simulink model "Simulation_Robotinos"  (R2017b)
settings: Solver=FixedStepAuto  StartTime=0.0  StopTime=100.0  FixedStep=0.005  RelTol=1e-3
InitFcn:
  | dt=0.005;
libraries: simulink x15
(part 3 of 4)

== matlab function Simulation_Robotinos/Bahnplanung2/Positionen_Robotinos_Filtern ==
  data: UDPDaten input; RobPos output; RobotinoID input; StoerPos output size=[1 15]; altePos input size=[1 15]; altePos1 output size=[1 15]
function [RobPos,StoerPos,altePos1]      = fcn(UDPDaten , RobotinoID, altePos)
StoerPos=zeros([1 15]);
RobPos=zeros([1 3]);
altePos1=zeros([1 15]);
%     case 5
%         RobPos(1:3) = UDPDaten(13:15);
%         StoerPos(1:12)=UDPDaten(1:12);
%Positionmerken
for x=0:4
    temp=abs(UDPDaten((x*3)+1:(x*3)+3));
    test=sum(temp);
    if(test==0)
     altePos1((x*3)+1:(x*3)+3)=altePos((x*3)+1:(x*3)+3);
    else
     altePos1((x*3)+1:(x*3)+3)=UDPDaten((x*3)+1:(x*3)+3);
    end
end

if RobotinoID==5
        RobPos(1:3) = altePos1(13:15);
        StoerPos(1:12)=altePos1(1:12);
    elseif RobotinoID == 4
        RobPos(1:3) = altePos1(10:12);
        StoerPos(1:9)=altePos1(1:9);
        StoerPos(10:12)=altePos1(13:15);
    elseif RobotinoID == 3
        RobPos(1:3) = altePos1(7:9);
        StoerPos(1:6)=altePos1(1:6);
        StoerPos(7:9)=altePos1(10:12);%      StoerPos(7:12)=UDPDaten(10:15);
        StoerPos(10:12)=altePos1(13:15);
    elseif RobotinoID == 2
        RobPos(1:3) = altePos1(4:6);
        StoerPos(1:3)=altePos1(1:3);
        StoerPos(4:9)=altePos1(7:12);%     StoerPos(4:12)=UDPDaten(7:15);
        StoerPos(10:12)=altePos1(13:15);
    elseif RobotinoID == 1
        RobPos(1:3) = altePos1(1:3);
        StoerPos(1:9)=altePos1(4:12);%     StoerPos(1:12)=UDPDaten(4:15);
        StoerPos(10:12)=altePos1(13:15);
        
end

== matlab function Simulation_Robotinos/Bahnplanung2/Status ==
  data: Fehler_IN input; Status_IN input; Status output
function Status       = fcn(Fehler_IN ,Status_IN)
if Fehler_IN > 0 
    Status = Fehler_IN + 4;
else
    Status = Status_IN;
end
end

== matlab function Simulation_Robotinos/Bahnplanung2/Trafo ==
  data: Vektor input; V_RobX output; Winkel input; V_RobY output
function [V_RobX, V_RobY]= fcn(Vektor,Winkel)
V_RobX=(cos(Winkel)*Vektor(1)+sin(Winkel)*Vektor(2));
V_RobY=(cos(Winkel)*Vektor(2)-sin(Winkel)*Vektor(1));

== matlab function Simulation_Robotinos/Bahnplanung2/Vektorberechnung/AusweichVektorBerechnung ==
  data: Zone input; ZielPos input; RobotinoPos input; Ausweichwert input; Vektor_In input; Vektor output
function Vektor  = fcn(Zone,ZielPos,RobotinoPos,Ausweichwert,Vektor_In)
Vektor=zeros([1 2]);
%Ausweichmanöver
Distanz=sqrt((RobotinoPos(1)-ZielPos(1))^2+(RobotinoPos(2)-ZielPos(2))^2);
K=1.4;
AVX=zeros([1 4]);
AVY=zeros([1 4]);
 for x=1:4
 AVX(x)=-K*Ausweichwert(2,x)*cos(Ausweichwert(1,x));
 AVY(x)=-K*Ausweichwert(2,x)*sin(Ausweichwert(1,x));
 end
if (Zone==0) && ((Distanz > 300)&&(RobotinoPos(2)> 500)&&(RobotinoPos(1)> 500))
 VektorX=Vektor_In(1)+sum(AVX);
 VektorY=Vektor_In(2)+sum(AVY);
else
 VektorX=Vektor_In(1);
 VektorY=Vektor_In(2);
end

%Bremsen vor dem Ziel

MaxDis=1000;
if Distanz > MaxDis
Vektor(1) = VektorX;
Vektor(2) = VektorY;
else
Vektor(1) = VektorX*Distanz/MaxDis;
Vektor(2) = VektorY*Distanz/MaxDis;  
end

end

== matlab function Simulation_Robotinos/Bahnplanung2/Vektorberechnung/Ausweichmanoever ==
  data: RobotinoPos input; StoerPos input; Vektor input; Ausweich output
function Ausweich  = fcn(RobotinoPos, StoerPos, Vektor)
Abstand=zeros([2 4]);
Ausweich=zeros([2 4]);%Zeile1 =Richtung(winkel in Rad) Zeile2=Intensität
for i=1:4
    Abstand(1,i)=-RobotinoPos(1)+StoerPos(1+((i-1)*3));
    Abstand(2,i)=-RobotinoPos(2)+StoerPos(2+((i-1)*3));
    Hyp=sqrt(Abstand(1,i)^2+Abstand(2,i)^2);
    if(Hyp==0)
        Hyp=1e-22;
    end
    if Hyp <=1000
        if Abstand(1,i) >= 0
             Ausweich(1,i)=+asin(Abstand(2,i)/Hyp)-pi/2;
        else
            Ausweich(1,i)=-asin(Abstand(2,i)/Hyp)+pi/2;
        end
        HypZiel=sqrt(Vektor(1)^2+Vektor(2)^2);
         if Vektor(1) >= 0
            Fahrwinkel=+asin(Vektor(2)/HypZiel);
        else
            Fahrwinkel=-asin(Vektor(2)/HypZiel)+pi;
        end
        if abs(Fahrwinkel-(Ausweich(1,i)+pi/2))<=pi
            if((Fahrwinkel-(Ausweich(1,i)+pi/2)) <= pi/6) && ((Fahrwinkel-(Ausweich(1,i)+pi/2))  >= -pi/6)
            Ausweich(2,i)=1;
             else
           Ausweich(2,i)=0; 
            end
        else
            if((2*pi)-abs(Fahrwinkel-(Ausweich(1,i)+pi/2)) <= pi/6) 
            Ausweich(2,i)=1;
             else
           Ausweich(2,i)=0; 
            end
        end
%         if (abs(Fahrwinkel)>pi/2) && (RobotinoPos(2)>1600)
%              if abs(Fahrwinkel-(Ausweich(1,i)+pi/2))<=pi
%             if((Fahrwinkel-(Ausweich(1,i)+pi/2)) <= pi/6) && ((Fahrwinkel-(Ausweich(1,i)+pi/2))  >= -pi/6)
%             Ausweich(2,i)=-0.5;
%              else
%            Ausweich(2,i)=0; 
%             end
%         else
%             if((2*pi)-abs(Fahrwinkel-(Ausweich(1,i)+pi/2)) <= pi/6) 
%             Ausweich(2,i)=-0.5;
%              else
%            Ausweich(2,i)=0; 
%             end
%         end
        %end
%         if (Vektor(2)~=0) && (sin(Ausweich(1,i)+pi/2)~=0)
%             Ausweich(2,i)=Vektor(2)/sin(Ausweich(1,i)+pi/2);
%         elseif (Vektor(1)~=0)&&(cos(Ausweich(1,i)+pi/2)~=0)
%              Ausweich(2,i)=Vektor(1)/cos(Ausweich(1,i)+pi/2);
%         else
%              Ausweich(2,i)=0;
%         end
    else
        Ausweich(1,i)=0;
        Ausweich(2,i)=0;
    end
    if StoerPos(2+((i-1)*3))<300
        Ausweich(2,i)=0;
    end
end

== matlab function Simulation_Robotinos/Bahnplanung2/Vektorberechnung/FahrendeRobotinosErkennen ==
  data: Stoerpos input; Robotinofaehrt output; Stoeralt input
function Robotinofaehrt = fcn(Stoerpos,Stoeralt)
Robotinofaehrt=zeros([1 4]);
for x=1:4
    if (abs(Stoeralt(1+(3*(x-1)))-Stoerpos(1+(3*(x-1)))) >= 10) && (abs(Stoeralt(2+(3*(x-1)))-Stoerpos(2+(3*(x-1)))) >= 10)
        Robotinofaehrt(x)=1;
    else
        Robotinofaehrt(x)=0;
    end
end

== matlab function Simulation_Robotinos/Bahnplanung2/Vektorberechnung/IR_Daten_Erfassen ==
  data: RobotinoDaten input; IRWerte output; RobPos input
function IRWerte = fcn(RobotinoDaten,RobPos)
IRWerte=zeros([2 9]);
IRDaten=zeros([1 9]);
IRDaten=RobotinoDaten(6:14);

for x=1:9
    if  (isnan(IRDaten(x))==0) && (IRDaten(x) <= 150)
    IRWerte(1,x)=cos(((x-1)*40*pi/180)+RobPos(3))*(IRDaten(x)+200)+RobPos(1);
    IRWerte(2,x)=sin(((x-1)*40*pi/180)+RobPos(3))*(IRDaten(x)+200)+RobPos(2);
    else
    IRWerte(1,x)=NaN;
    IRWerte(2,x)=NaN;
    end
end

== matlab function Simulation_Robotinos/Bahnplanung2/Vektorberechnung/Vektorberechnung ==
  data: StoerPos input; IRWerte input; RobotinoPos input; RobotinoFaehrt input; ZielPos input; Vektor output; Zone output; AlteZone input
function [Vektor,Zone] = fcn( StoerPos, IRWerte,RobotinoPos,RobotinoFaehrt,ZielPos,AlteZone)
Stationen=[1103,2308,3507,4694,6300,6300;
            2832,2832,2832,2832,2608,3085;];
Vektor=zeros([1 2]);
%Stationen Einflussvektor
K=500;
sigma=187;
SVX=zeros([1 6]);
SVY=zeros([1 6]);
for x=1:4 %%Stationspotentiale
SVX(x)= -K*exp(-((RobotinoPos(1)-Stationen(1,x))^2+(RobotinoPos(2)-Stationen(2,x))^2)/(2*(sigma^2)))*((RobotinoPos(1)-Stationen(1,x))/(sigma^2));
SVY(x)= -K*exp(-((RobotinoPos(1)-Stationen(1,x))^2+(RobotinoPos(2)-Stationen(2,x))^2)/(2*(sigma^2)))*((RobotinoPos(2)-Stationen(2,x))/(sigma^2));
end
K=300;
sigma=100; %% mal schauen ob so gut
for x=5:6 %% Ladestation
SVX(x)= -K*exp(-((RobotinoPos(1)-Stationen(1,x))^2+(RobotinoPos(2)-Stationen(2,x))^2)/(2*(sigma^2)))*((RobotinoPos(1)-Stationen(1,x))/(sigma^2));
SVY(x)= -K*exp(-((RobotinoPos(1)-Stationen(1,x))^2+(RobotinoPos(2)-Stationen(2,x))^2)/(2*(sigma^2)))*((RobotinoPos(2)-Stationen(2,x))/(sigma^2));
end
%Zielvektor
K=0.7;%=0.5;
if (RobotinoPos(1)~=ZielPos(1)) && (RobotinoPos(2)~=ZielPos(2))  %%Ziel
    ZVX = K*(RobotinoPos(1)-ZielPos(1))/sqrt((RobotinoPos(1)-ZielPos(1))^2 +(RobotinoPos(2)-ZielPos(2))^2);
    ZVY = K*(RobotinoPos(2)-ZielPos(2))/sqrt((RobotinoPos(1)-ZielPos(1))^2 +(RobotinoPos(2)-ZielPos(2))^2);
else
    ZVX=0;
    ZVY=0;
end

%Robtino Stoervektoren
%K=25 im Fifo

RVX=zeros([1 4]);
RVY=zeros([1 4]);
for x=1:4
if (RobotinoFaehrt(x) == 1) && (RobotinoPos(2)> 500)
K=1300;%K=1000;
sigma=240;
elseif (RobotinoPos(2)> 2500)
K=700;%500
sigma=200;
elseif (RobotinoPos(2)< 2500)
K=1000;%700
sigma=200;
end
RVX(x)=-K*exp(-((RobotinoPos(1)-StoerPos((x*3)-2))^2+(RobotinoPos(2)-StoerPos((x*3)-1))^2)/(2*(sigma^2)))*((RobotinoPos(1)-StoerPos((x*3)-2))/(sigma^2));
RVY(x)=-K*exp(-((RobotinoPos(1)-StoerPos((x*3)-2))^2+(RobotinoPos(2)-StoerPos((x*3)-1))^2)/(2*(sigma^2)))*((RobotinoPos(2)-StoerPos((x*3)-1))/(sigma^2));
end

%Infrarot Einflussvektor
K=600;%500;
sigma=250;
IRVX=zeros([1 9]);
IRVY=zeros([1 9]);
for x=1:9
    if(isnan(IRWerte(1,x))==0)||(isnan(IRWerte(2,x))==0)
       if (RobotinoPos(2)> 500)
    IRVX(x)=-K*exp(-((RobotinoPos(1)-IRWerte(1,x))^2+(RobotinoPos(2)-IRWerte(2,x))^2)/(2*(sigma^2)))*((RobotinoPos(1)-IRWerte(1,x))/(sigma^2));
    IRVY(x)=-K*exp(-((RobotinoPos(1)-IRWerte(1,x))^2+(RobotinoPos(2)-IRWerte(2,x))^2)/(2*(sigma^2)))*((RobotinoPos(2)-IRWerte(2,x))/(sigma^2));
       else
    IRVX=0;
    IRVY=0;
       end
    else
    IRVX(x)=0;
    IRVY(x)=0;
    end
end


 
K=0.4; %Steigung der schrägen
x=RobotinoPos(1);
y=RobotinoPos(2);
x_test=0;
y_test=0;
VektorX=0;
VektorY=0;
%% Einteilung des Vektorbereichs in verschidene Zonen
%%Einbahnstraßen hinter und neben den Stationen
 if (x >601) && (x<=5301) && (y>2501) && (y<=3201)
    Zone=4;
elseif (x >2751) && (x<=5501) && (y>3201)
    Zone=1;
elseif (x > 601) && (x<=2751) && (y>3201)
    Zone=2;
 elseif (x<=601) && (y>2001)%% y auf 2001 von 2501
     Zone=3;  
 elseif (x >5001) && (y>2501) && (AlteZone==1 || AlteZone==5)
     Zone=5;
 else
     Zone=0;
 end

KE=1000;
sigma=50;
Parabel=1000;
 if Zone == 0 % Fahrbereich
     if (x <= 5500) && (y <= 2500)
         x_test=(1/sigma)*KE*exp(-x/sigma);
         y_test=(-1/sigma)*KE*exp((y-2500)/sigma);
     elseif (x > 5500) && (y <= 2500)
         x_test=(1/sigma)*KE*exp((-(x-5500)+(y-2500))/sigma);
         y_test=(-1/sigma)*KE*exp((-(x-5500)+(y-2500))/sigma);
     elseif (x > 5500) && (y > 2500)
         x_test=(1/sigma)*KE*exp(-(x-5500)/sigma);
         y_test=(-1/sigma)*KE*exp((y-3600)/sigma);
     end
 MVX=x_test+(-1/sigma)*KE*exp((x-7400)/sigma);
 MVY=y_test+(1/sigma)*KE*exp(-y/sigma);
 
 VektorX=sum(SVX(5:6))+sum(RVX)+ZVX+sum(IRVX)-MVX;
 VektorY=sum(SVY(5:6))+sum(RVY)+ZVY+sum(IRVY)-MVY;
 elseif Zone == 1 %Rinne nach rechts weg
     MVX=K; %Konstante Steigung
     MVY=-2*(y-3500)/Parabel; % Parabel abgeleitet
 VektorX=sum(RVX)-MVX;
 VektorY=sum(RVY)-MVY;
 elseif Zone == 2 %Rinne nach links weg
     MVX=-K; %Konstante Steigung
     MVY=-2*(y-3500)/Parabel; % Parabel abgeleitet
      VektorX=sum(RVX)-MVX;
      VektorY=sum(RVY)-MVY;
 elseif Zone == 3 %Rinne nach unten weg
     MVX=-2*(x-300)/Parabel; %Konstante Steigung
     MVY=-K; % Parabel abgeleitet
     VektorX=sum(RVX)+sum(IRVX)-MVX;
     VektorY=sum(RVY)+sum(IRVY)-MVY;
 elseif Zone == 5 %Rinne vorne weg
     MVX=-2*(x-5500)/Parabel; %Konstante Steigung
     MVY=-K; % Parabel abgeleitet
     VektorX=sum(RVX)+sum(IRVX)-MVX;
     VektorY=sum(RVY)+sum(IRVY)-MVY;
 else 
     MVX=0;
     MVY=K;
      VektorX=sum(RVX)+sum(SVX(1:4))-MVX;
      VektorY=sum(RVY)+sum(SVY(1:4))-MVY;
 end  
      Vektor(1)=VektorX;
      Vektor(2)=VektorY;
 end

== matlab function Simulation_Robotinos/Bahnplanung2/Vektorbrbegrenzungberchnen1 ==
  data: Vektor_In input; IRDaten input; Vektor output; Transportbereich_aktiv input; RobPos input; FilterIN input; Filter output
function [Vektor,Filter] = fcn(Vektor_In,IRDaten,Transportbereich_aktiv,RobPos,FilterIN)
Vektor=zeros([1 2]);
Filter=zeros([10 2]);
if (Transportbereich_aktiv==1) && (RobPos(1)>=0) && (RobPos(2)>=0)
    

 Filter(1,1)=Vektor_In(1);
 Filter(1,2)=Vektor_In(2);
 for x=1:9
     Filter(x+1,1)=FilterIN(x,1);
     Filter(x+1,2)=FilterIN(x,2);     
 end
 Vektor(1) =sum(Filter(:,1))/10;
 Vektor(2) =sum(Filter(:,2))/10;
 
 %Vektor(1) = Vektor_In(1);
 %Vektor(2) = Vektor_In(2);
 for x=1:9
if  (isnan(IRDaten(1,x))==0) && (IRDaten(1,x) <= 150)
    for x=1:2
    K=0.1; %Begrenzung langsame Zone
        if  Vektor(x)> K
            Vektor(x) = K;
        elseif Vektor(x) <-K
            Vektor(x)=-K;
        end
    end
end
 end
if (RobPos(2)<500)||(RobPos(2)>2300)
    for x=1:2
    K=0.3; %Begrenzung langsame Zone
        if  Vektor(x)> K
            Vektor(x) = K;
        elseif Vektor(x) <-K
            Vektor(x)=-K;
        end
    end
else
    for x=1:2
    K=0.7; %Begrenzung schnelle Zone
        if  Vektor(x)> K
            Vektor(x) = K;
        elseif Vektor(x) <-K
            Vektor(x)=-K;
        end
    end
end
end

== stateflow chart Simulation_Robotinos/Bahnplanung3/Auftrags_Koordination ==
  settings: updateMethod=DISCRETE  sampleTime=dt
  state Auftragskoordination
    state WerkstueckAufgenommen
      entry:Werkstueck=1,
      AktuellesZiel=ZielPos,
      Bearbeitet=1;
    state WerkstueckAbgelegt
      entry:Werkstueck=0,
      AktuellesZiel=ZielPos,
      Bearbeitet=1;
    state KeinWerkstueckAufgenommen
      entry:Werkstueck=0,
      AktuellesZiel=WerkstueckPos,
      Bearbeitet=1;
    state AufAuftragWarten
      entry:Werkstueck=0,
      AktuellesZiel=100
      Bearbeitet=0;
    state Laden
      entry:Werkstueck=0,
      AktuellesZiel=90,
      Bearbeitet=1;
    state Ladenabgeschlossen
      entry:Werkstueck=0,
      AktuellesZiel=90,
      Bearbeitet=1;
    WerkstueckAufgenommen -> WerkstueckAufgenommen [order 1] : [Fehler==3]
    WerkstueckAufgenommen -> WerkstueckAbgelegt [order 3] : [Werkstueckerkannt==0 && Transportbereich==0]
    KeinWerkstueckAufgenommen -> WerkstueckAufgenommen [order 1] : [Werkstueckerkannt==1 && Transportbereich==1]
    WerkstueckAufgenommen -> AufAuftragWarten [order 2] : [Fehler==2  && Transportbereich==1]
    (default) -> AufAuftragWarten
    WerkstueckAbgelegt -> AufAuftragWarten : [Werkstueckerkannt==0 && Transportbereich==1]
    KeinWerkstueckAufgenommen -> AufAuftragWarten [order 2] : [Fehler==1&& Transportbereich==1]
    AufAuftragWarten -> KeinWerkstueckAufgenommen [order 1] : [NeuerAuftrag ==1 && WerkstueckPos< 80 && Fehler==0]
    AufAuftragWarten -> Laden [order 2] : [NeuerAuftrag ==1 && WerkstueckPos>= 80]
    Ladenabgeschlossen -> AufAuftragWarten : [Transportbereich==1]
    Laden -> Ladenabgeschlossen : [Status==4]
  data: NeuerAuftrag input; WerkstueckPos input; ZielPos input; AktuellesZiel output; Werkstueck output; Werkstueckerkannt input; Transportbereich input; Bearbeitet output; Status input; Fehler input

== matlab function Simulation_Robotinos/Bahnplanung3/Fehler_Merker ==
  data: Fehler_IN input; Reset input; Transportbereich input; Werkstueckerkannt input; Werkstueck input; Fehler_OUT output; Fehler_alt input
function Fehler_OUT       = fcn(Fehler_IN ,Reset, Transportbereich, Werkstueckerkannt,Werkstueck, Fehler_alt)
if Reset == 1 || Fehler_IN ~= 0
    Fehler_OUT=Fehler_IN;
else
    if Transportbereich == 1 && Werkstueckerkannt~=1 && Werkstueck == 1
        Fehler_OUT = 2;
    else
       Fehler_OUT=Fehler_alt; 
    end 
end
end

== stateflow chart Simulation_Robotinos/Bahnplanung3/Fifo Steuerung/Fifo ==
  settings: updateMethod=DISCRETE  sampleTime=dt
  state FIFOStationen
    state Auftrag_Roboter_1
    state Zielbereich_untersuchen
      entry:
      ersterFifo=floor(Zielstation/2)*3+2*mod(Zielstation,2)+1;
    state Fifo_doppelt_besetzt
      entry:
      dritterFifo=floor(Zielstation/2)*3+2-2*mod(Zielstation,2)+1,
      Fifo=3;
    state Fifo_einfachbesetzt1
      entry:
      zweiterFifo=floor(Zielstation/2)*3+1+1,
      Fifo=2;
    state Fifo_voll
      entry:
      Fifo=4;
    state Fifo_frei
      entry:
      Fifo=1;
    state Uebergabepunkt_gleich_Zielpunkt
      entry:
      Fifo=0;
    (default) -> Auftrag_Roboter_1
    Auftrag_Roboter_1 -> Zielbereich_untersuchen : [Zielposition>-1]
    Zielbereich_untersuchen -> Fifo_einfachbesetzt1 [order 1] : [(FifoArray(ersterFifo)~=0)| (FifoArray(ersterFifo)==0 & StationArray(Zielstation+1)~=0) ]
    Uebergabepunkt_gleich_Zielpunkt -> Zielbereich_untersuchen
    Zielbereich_untersuchen -> Uebergabepunkt_gleich_Zielpunkt [order 2]
    Fifo_einfachbesetzt1 -> Fifo_doppelt_besetzt [order 1] : [(FifoArray(zweiterFifo)~=0)]
    Fifo_doppelt_besetzt -> Fifo_voll [order 2] : [(FifoArray(dritterFifo)~=0)]
    Fifo_einfachbesetzt1 -> Fifo_frei [order 2] : [FifoArray(ersterFifo)==0]
    Fifo_frei -> Uebergabepunkt_gleich_Zielpunkt : [ StationArray(Zielstation+1)==0]
    Fifo_doppelt_besetzt -> Fifo_einfachbesetzt1 [order 1] : [FifoArray(zweiterFifo)==0]
    Fifo_voll -> Fifo_doppelt_besetzt : [FifoArray(dritterFifo)==0]
  state Wartebereich
    entry: Fifo=4;
  state Ladestation
    entry: Fifo=0;
  state Ladestation1
    entry: Fifo=4;
  FIFOStationen -> FIFOStationen [order 1] : [after(10000, tick)]
  (default) -> Wartebereich
  Wartebereich -> FIFOStationen [order 1] : [Zielstation<8]
  FIFOStationen -> Wartebereich [order 2] : [Zielstation==10]
  Ladestation -> Wartebereich [order 1] : [Zielstation==10]
  Wartebereich -> Ladestation [order 2] : [Zielstation>=8 & Zielstation<10]
  Ladestation -> FIFOStationen [order 2] : [Zielstation<8]
  FIFOStationen -> Ladestation [order 3] : [Zielstation>=8 & Zielstation<10]
  Ladestation -> Ladestation1 [order 3] : [Ladenarray(1)~=0]
  Ladestation1 -> Ladestation : [Ladenarray(1)==0]
  data: FifoArray input; Zielposition input; Zielstation input; Fifo output; StationArray input; dritterFifo local; zweiterFifo local; ersterFifo local; Ladenarray input

== matlab function Simulation_Robotinos/Bahnplanung3/Fifo Steuerung/Globale Markierung1 ==
  data: StationArray1 output; Robbi input; FifoArray input; FifoArray1 output; LadeArray1 output; LadeArray input
function [StationArray1,FifoArray1,LadeArray1]= fcn(Robbi,FifoArray,LadeArray)
X=zeros([1 4]);
Y=zeros([1 4]);
X=[Robbi(1) Robbi(4) Robbi(7) Robbi(10)];
Y=[Robbi(2) Robbi(5) Robbi(8) Robbi(11)];
FifoArray1=zeros([1 12]);
FifoArray1=FifoArray(1:12);
StationArray1=zeros([1 8]);
LadeArray1=zeros([1 2]);
LadeArray1=LadeArray(1:2);
N=zeros([1 4]);
S=zeros([1 4]);
L=zeros([1 4]);
  for n= 1 : 1 : 4
    L(n)=round((Y(n)-2592)/500)+1;
    N(n)=round((X(n)-703)/425)+1;   % Berechnung in welchem Fifo der Roboter sich befindet
    S(n)=round((X(n)-900)/560)+1;   %Berechnung in welcher Station der Roboter sich befindet
     if (X(n)<=6000 || X(n)>6500)
        for i=1:2
            if LadeArray1(i)==n
                LadeArray1(i)=0;
            end
        end
     end
    if (X(n)>6000 && X(n)<=6500 && Y(n)>2300 && Y(n)<=3300 && L(n)<=2 && L(n)>0)
        LadeArray1(1)=n;
        LadeArray1(2)=n;
    end  
   
    for i=1:8
          if StationArray1(i)==n
                StationArray1(i)=0;
          end
    end
    if (Y(n)>2000 && Y(n)<3300 && X(n)<5100 && S(n)<=8 && S(n)>0) %% Setzen der Stationspos.
         for i=1:12
            if FifoArray1(i)==n
                FifoArray1(i)=0;
            end
         end
       
        StationArray1(S(n))=n;
    end
    if (Y(n)<450 && X(n)>100 && X(n)<6000 && N(n)<=12 && N(n)>0) %% Setzten der aktuellen Fifo Pos
        for i=1:12
            if FifoArray1(i)==n
                FifoArray1(i)=0;
            end
        end
            FifoArray1(N(n))=n;
    end  
    if (X(n)>6000 && Y(n)<2000)%%Rücksetzen de4r FIFOs auf Warteposition
        for i=1:12
            if FifoArray1(i)==n
                FifoArray1(i)=0;
            end
        end
    end
  end
end

== matlab function Simulation_Robotinos/Bahnplanung3/Fifo Steuerung/Positionszuweisung ==
  data: Fifo input; Zielstation input; Endposition output; RoboterID input
function Endposition = fcn(Fifo,Zielstation,RoboterID)
Endposition=zeros([1 2]);

WartepositionX= [6200 6800 7200 7200 7200]; %[7200 6800 7200 6200 7200];
WartepositionY= [250 250 550 1150 1750];    %[550 250 1150 250 1750];

StationvorneX=[853 1361 2058 2559 3256 3762 4448 4953 5965 5965];
StationvorneY=[2300 2300 2300 2300 2300 2300 2300 2300 3080 2593];
%Stationhinten=[856 1364 2059 2560 3259 3763 4451 4958];

ersterFifo=floor(Zielstation/2)*3+2*mod(Zielstation,2);
zweiterFifo=floor(Zielstation/2)*3+1;
dritterFifo=floor(Zielstation/2)*3+2-2*mod(Zielstation,2);

if Fifo==0
    Endposition(1)=StationvorneX(Zielstation+1);
    Endposition(2)=StationvorneY(Zielstation+1);
    else if Fifo==1
        Endposition(1)= ersterFifo*425+703;
        Endposition(2)= 250;
       
    else if Fifo==2
            Endposition(1)= zweiterFifo*425+703;
            Endposition(2)= 250;
        
    else if Fifo==3
            Endposition(1)= dritterFifo*425+703;
            Endposition(2)= 250;
            else
            Endposition(2)= WartepositionY(RoboterID);
            Endposition(1)= WartepositionX(RoboterID);
        end
        end
        end
end
end

== matlab function Simulation_Robotinos/Bahnplanung3/Fifo Steuerung/ZielPosSplitten ==
  data: AktuellesZiel input; ZielPos output; Zielstation output
function [ZielPos,Zielstation]= fcn(AktuellesZiel)
ZielPos=mod(AktuellesZiel,10);
Zielstation=round(AktuellesZiel/10);

== matlab function Simulation_Robotinos/Bahnplanung3/Fifo Steuerung/ZielStation_Erreicht ==
  data: Erreicht output; AktuellePos input; Zielpos input
function Erreicht = fcn(AktuellePos,Zielpos)
Abstand=sqrt((AktuellePos(1)-Zielpos(1))^2+(AktuellePos(2)-Zielpos(2))^2);
%S=round((X-900)/560);
if AktuellePos(2) >2000 && Abstand < 150
    Erreicht=1;
else
    Erreicht=0;
end
end

== stateflow chart Simulation_Robotinos/Bahnplanung3/Kommunikation_mit_GW1_3 ==
  settings: updateMethod=DISCRETE  sampleTime=dt
  state KommunikationGW3
    state Fertigungsbereich
      entry:Transportbereich=0,
      Fertigungsbereich=1;
      state RFID_einchecken
        entry:Zielposition=Ziel-mod(Ziel,10)+3,
        Aktion_an_Position=Aktion_Warten,
        Status=2;
      state Startpunkt
        entry: Zielposition=Ziel-mod(Ziel,10);
        Aktion_an_Position=Aktion_Warten,
        Status=1;
      state Warten
        during: Bereich_Verlassen=1,
      state Bereich_verlassen_hinten
        entry:Zielposition=Ziel-mod(Ziel,10)+4,
        Aktion_an_Position=Aktion_Warten,
        Status=1;
      state Bereich_verlassen_vorne1
        entry:Zielposition=Ziel-mod(Ziel,10),
        Aktion_an_Position=Aktion_Warten,
        Status=1;
      state Warten1
      state Bereich_verlassen
        entry:
        ersterFifo=floor(floor(Ziel/10)/2)*3+2*mod(floor(Ziel/10),2)+1;
        Aktion_an_Position=Aktion_Warten,
      state Position_anfahren
        entry:Zielposition=Ziel,
        Status=1,
        if Werkstueck==0
        Aktion_an_Position=Aktion_Aufnehmen;
        else
        Aktion_an_Position=Aktion_Ablegen;
        end
      state RFID_auschecken
        entry:Zielposition=Ziel-mod(Ziel,10)+3,
        Aktion_an_Position=Aktion_Warten,
        Status=3;
      state Warten2
      Startpunkt -> Startpunkt [order 1] : [Fehler==3]
      (default) -> Startpunkt
      Startpunkt -> RFID_einchecken [order 2] : [Ziel_anfordern==1 & Werkstueck==1]
      Position_anfahren -> Startpunkt [order 3] : [Fehler==3 & Ziel_anfordern==1]
      Startpunkt -> Position_anfahren [order 3] : [Ziel_anfordern==1 & Werkstueck==0]
      RFID_einchecken -> Warten1 : [Ziel_anfordern==1 ]
      Bereich_verlassen_hinten -> Warten : [Ziel_anfordern==1]
      Bereich_verlassen_vorne1 -> Warten : [Ziel_anfordern==1]
      Warten1 -> Position_anfahren : [RFID_Anmeldung==1]
      Bereich_verlassen -> Bereich_verlassen_hinten [order 2]
      Bereich_verlassen -> Bereich_verlassen_vorne1 [order 1] : [FifoArray(ersterFifo)==0]
      Position_anfahren -> Bereich_verlassen [order 2] : [Fehler==1 & Ziel_anfordern==1]
      Position_anfahren -> Bereich_verlassen [order 1] : [Ziel_anfordern==1 & (Aktion_an_Position==Aktion_Ablegen)]
      Warten2 -> Bereich_verlassen : [RFID_Abmeldung==1]
      Position_anfahren -> RFID_auschecken [order 4] : [Ziel_anfordern==1 & (Aktion_an_Position==Aktion_Aufnehmen) & Fehler==0]
      RFID_auschecken -> Warten2 : [Ziel_anfordern==1]
    state Ladestationanfahren2
      entry: Zielposition=100,
      Transportbereich=0,
      Fertigungsbereich=1,
      Status=1;
    state Transportbereich
      entry:Transportbereich=1,
      Zielposition=999,
      Fertigungsbereich=0,
      Bereich_Verlassen=0,
      Geladen=0,
      Status=1;
    state Warten3
    state Ladestationanfahren1
      entry: Zielposition=80,
      Transportbereich=0,
      Fertigungsbereich=1,
      Status=1;
    state Laden4
      entry: Zielposition=110,
      Transportbereich=0,
      Fertigungsbereich=1,
      Geladen=1,
      Status=4;
    state Laden2
      entry: Zielposition=110,
      Transportbereich=0,
      Fertigungsbereich=1,
      Status=1;
    state Laden1
      entry: Zielposition=90,
      Transportbereich=0,
      Fertigungsbereich=1,
      Status=1;
    state Laden3
      entry: Zielposition=90,
      Transportbereich=0,
      Fertigungsbereich=1,
      Geladen =1,
      Status=4;
    (default) -> Transportbereich
    Ladestationanfahren2 -> Transportbereich [order 2] : [ Geladen==1 & Ziel_anfordern==1 ]
    Transportbereich -> Fertigungsbereich [order 1] : [(ZielStation_Erreicht==1) & (floor(Ziel/10)<=7)]
    Transportbereich -> Ladestationanfahren2 [order 2] : [(ZielStation_Erreicht==1) & (floor(Ziel/10)==9)]
    Warten3 -> Transportbereich
    Fertigungsbereich -> Warten3 : [Bereich_Verlassen==1]
    Ladestationanfahren2 -> Laden2 [order 1] : [ Geladen==0 & Ziel_anfordern==1 ]
    Laden4 -> Ladestationanfahren2 : [Ladenabgeschlossen==1 ]
    Transportbereich -> Ladestationanfahren1 [order 3] : [(ZielStation_Erreicht==1) & (floor(Ziel/10)==8)]
    Ladestationanfahren1 -> Transportbereich [order 2] : [ Geladen==1 & Ziel_anfordern==1 ]
    Ladestationanfahren1 -> Laden1 [order 1] : [ Geladen==0 & Ziel_anfordern==1 ]
    Laden3 -> Ladestationanfahren1 : [Ladenabgeschlossen==1 ]
    Laden2 -> Laden4 : [Ziel_anfordern==1 ]
    Laden1 -> Laden3 : [Ziel_anfordern==1 ]
  data: Transportbereich output; Fertigungsbereich output; Ziel input; Zielposition output; Aktion_an_Position output double; Aktion_Warten local double =0; Aktion_Aufnehmen local double =1; Aktion_Ablegen local double =2; Werkstueck input double; Bereich_Verlassen local; Status output; FifoArray input; ersterFifo local double; Ziel_anfordern input; ZielStation_Erreicht input double; RFID_Anmeldung input; RFID_Abmeldung input; Ladenabgeschlossen input; Geladen local; Fehler input

== matlab function Simulation_Robotinos/Bahnplanung3/Positionen_Robotinos_Filtern ==
  data: UDPDaten input; RobPos output; RobotinoID input; StoerPos output size=[1 15]; altePos input size=[1 15]; altePos1 output size=[1 15]
function [RobPos,StoerPos,altePos1]      = fcn(UDPDaten , RobotinoID, altePos)
StoerPos=zeros([1 15]);
RobPos=zeros([1 3]);
altePos1=zeros([1 15]);
%     case 5
%         RobPos(1:3) = UDPDaten(13:15);
%         StoerPos(1:12)=UDPDaten(1:12);
%Positionmerken
for x=0:4
    temp=abs(UDPDaten((x*3)+1:(x*3)+3));
    test=sum(temp);
    if(test==0)
     altePos1((x*3)+1:(x*3)+3)=altePos((x*3)+1:(x*3)+3);
    else
     altePos1((x*3)+1:(x*3)+3)=UDPDaten((x*3)+1:(x*3)+3);
    end
end

if RobotinoID==5
        RobPos(1:3) = altePos1(13:15);
        StoerPos(1:12)=altePos1(1:12);
    elseif RobotinoID == 4
        RobPos(1:3) = altePos1(10:12);
        StoerPos(1:9)=altePos1(1:9);
        StoerPos(10:12)=altePos1(13:15);
    elseif RobotinoID == 3
        RobPos(1:3) = altePos1(7:9);
        StoerPos(1:6)=altePos1(1:6);
        StoerPos(7:9)=altePos1(10:12);%      StoerPos(7:12)=UDPDaten(10:15);
        StoerPos(10:12)=altePos1(13:15);
    elseif RobotinoID == 2
        RobPos(1:3) = altePos1(4:6);
        StoerPos(1:3)=altePos1(1:3);
        StoerPos(4:9)=altePos1(7:12);%     StoerPos(4:12)=UDPDaten(7:15);
        StoerPos(10:12)=altePos1(13:15);
    elseif RobotinoID == 1
        RobPos(1:3) = altePos1(1:3);
        StoerPos(1:9)=altePos1(4:12);%     StoerPos(1:12)=UDPDaten(4:15);
        StoerPos(10:12)=altePos1(13:15);
        
end

== matlab function Simulation_Robotinos/Bahnplanung3/Status ==
  data: Fehler_IN input; Status_IN input; Status output
function Status       = fcn(Fehler_IN ,Status_IN)
if Fehler_IN > 0 
    Status = Fehler_IN + 4;
else
    Status = Status_IN;
end
end

== matlab function Simulation_Robotinos/Bahnplanung3/Trafo ==
  data: Vektor input; V_RobX output; Winkel input; V_RobY output
function [V_RobX, V_RobY]= fcn(Vektor,Winkel)
V_RobX=(cos(Winkel)*Vektor(1)+sin(Winkel)*Vektor(2));
V_RobY=(cos(Winkel)*Vektor(2)-sin(Winkel)*Vektor(1));

== matlab function Simulation_Robotinos/Bahnplanung3/Vektorberechnung/AusweichVektorBerechnung ==
  data: Zone input; ZielPos input; RobotinoPos input; Ausweichwert input; Vektor_In input; Vektor output
function Vektor  = fcn(Zone,ZielPos,RobotinoPos,Ausweichwert,Vektor_In)
Vektor=zeros([1 2]);
%Ausweichmanöver
Distanz=sqrt((RobotinoPos(1)-ZielPos(1))^2+(RobotinoPos(2)-ZielPos(2))^2);
K=1.4;
AVX=zeros([1 4]);
AVY=zeros([1 4]);
 for x=1:4
 AVX(x)=-K*Ausweichwert(2,x)*cos(Ausweichwert(1,x));
 AVY(x)=-K*Ausweichwert(2,x)*sin(Ausweichwert(1,x));
 end
if (Zone==0) && ((Distanz > 300)&&(RobotinoPos(2)> 500)&&(RobotinoPos(1)> 500))
 VektorX=Vektor_In(1)+sum(AVX);
 VektorY=Vektor_In(2)+sum(AVY);
else
 VektorX=Vektor_In(1);
 VektorY=Vektor_In(2);
end

%Bremsen vor dem Ziel

MaxDis=1000;
if Distanz > MaxDis
Vektor(1) = VektorX;
Vektor(2) = VektorY;
else
Vektor(1) = VektorX*Distanz/MaxDis;
Vektor(2) = VektorY*Distanz/MaxDis;  
end

end

== matlab function Simulation_Robotinos/Bahnplanung3/Vektorberechnung/Ausweichmanoever ==
  data: RobotinoPos input; StoerPos input; Vektor input; Ausweich output
function Ausweich  = fcn(RobotinoPos, StoerPos, Vektor)
Abstand=zeros([2 4]);
Ausweich=zeros([2 4]);%Zeile1 =Richtung(winkel in Rad) Zeile2=Intensität
for i=1:4
    Abstand(1,i)=-RobotinoPos(1)+StoerPos(1+((i-1)*3));
    Abstand(2,i)=-RobotinoPos(2)+StoerPos(2+((i-1)*3));
    Hyp=sqrt(Abstand(1,i)^2+Abstand(2,i)^2);
    if(Hyp==0)
        Hyp=1e-22;
    end
    if Hyp <=1000
        if Abstand(1,i) >= 0
             Ausweich(1,i)=+asin(Abstand(2,i)/Hyp)-pi/2;
        else
            Ausweich(1,i)=-asin(Abstand(2,i)/Hyp)+pi/2;
        end
        HypZiel=sqrt(Vektor(1)^2+Vektor(2)^2);
         if Vektor(1) >= 0
            Fahrwinkel=+asin(Vektor(2)/HypZiel);
        else
            Fahrwinkel=-asin(Vektor(2)/HypZiel)+pi;
        end
        if abs(Fahrwinkel-(Ausweich(1,i)+pi/2))<=pi
            if((Fahrwinkel-(Ausweich(1,i)+pi/2)) <= pi/6) && ((Fahrwinkel-(Ausweich(1,i)+pi/2))  >= -pi/6)
            Ausweich(2,i)=1;
             else
           Ausweich(2,i)=0; 
            end
        else
            if((2*pi)-abs(Fahrwinkel-(Ausweich(1,i)+pi/2)) <= pi/6) 
            Ausweich(2,i)=1;
             else
           Ausweich(2,i)=0; 
            end
        end
%         if (abs(Fahrwinkel)>pi/2) && (RobotinoPos(2)>1600)
%              if abs(Fahrwinkel-(Ausweich(1,i)+pi/2))<=pi
%             if((Fahrwinkel-(Ausweich(1,i)+pi/2)) <= pi/6) && ((Fahrwinkel-(Ausweich(1,i)+pi/2))  >= -pi/6)
%             Ausweich(2,i)=-0.5;
%              else
%            Ausweich(2,i)=0; 
%             end
%         else
%             if((2*pi)-abs(Fahrwinkel-(Ausweich(1,i)+pi/2)) <= pi/6) 
%             Ausweich(2,i)=-0.5;
%              else
%            Ausweich(2,i)=0; 
%             end
%         end
        %end
%         if (Vektor(2)~=0) && (sin(Ausweich(1,i)+pi/2)~=0)
%             Ausweich(2,i)=Vektor(2)/sin(Ausweich(1,i)+pi/2);
%         elseif (Vektor(1)~=0)&&(cos(Ausweich(1,i)+pi/2)~=0)
%              Ausweich(2,i)=Vektor(1)/cos(Ausweich(1,i)+pi/2);
%         else
%              Ausweich(2,i)=0;
%         end
    else
        Ausweich(1,i)=0;
        Ausweich(2,i)=0;
    end
    if StoerPos(2+((i-1)*3))<300
        Ausweich(2,i)=0;
    end
end

== matlab function Simulation_Robotinos/Bahnplanung3/Vektorberechnung/FahrendeRobotinosErkennen ==
  data: Stoerpos input; Robotinofaehrt output; Stoeralt input
function Robotinofaehrt = fcn(Stoerpos,Stoeralt)
Robotinofaehrt=zeros([1 4]);
for x=1:4
    if (abs(Stoeralt(1+(3*(x-1)))-Stoerpos(1+(3*(x-1)))) >= 10) && (abs(Stoeralt(2+(3*(x-1)))-Stoerpos(2+(3*(x-1)))) >= 10)
        Robotinofaehrt(x)=1;
    else
        Robotinofaehrt(x)=0;
    end
end

== matlab function Simulation_Robotinos/Bahnplanung3/Vektorberechnung/IR_Daten_Erfassen ==
  data: RobotinoDaten input; IRWerte output; RobPos input
function IRWerte = fcn(RobotinoDaten,RobPos)
IRWerte=zeros([2 9]);
IRDaten=zeros([1 9]);
IRDaten=RobotinoDaten(6:14);

for x=1:9
    if  (isnan(IRDaten(x))==0) && (IRDaten(x) <= 150)
    IRWerte(1,x)=cos(((x-1)*40*pi/180)+RobPos(3))*(IRDaten(x)+200)+RobPos(1);
    IRWerte(2,x)=sin(((x-1)*40*pi/180)+RobPos(3))*(IRDaten(x)+200)+RobPos(2);
    else
    IRWerte(1,x)=NaN;
    IRWerte(2,x)=NaN;
    end
end

== matlab function Simulation_Robotinos/Bahnplanung3/Vektorberechnung/Vektorberechnung ==
  data: StoerPos input; IRWerte input; RobotinoPos input; RobotinoFaehrt input; ZielPos input; Vektor output; Zone output; AlteZone input
function [Vektor,Zone] = fcn( StoerPos, IRWerte,RobotinoPos,RobotinoFaehrt,ZielPos,AlteZone)
Stationen=[1103,2308,3507,4694,6300,6300;
            2832,2832,2832,2832,2608,3085;];
Vektor=zeros([1 2]);
%Stationen Einflussvektor
K=500;
sigma=187;
SVX=zeros([1 6]);
SVY=zeros([1 6]);
for x=1:4 %%Stationspotentiale
SVX(x)= -K*exp(-((RobotinoPos(1)-Stationen(1,x))^2+(RobotinoPos(2)-Stationen(2,x))^2)/(2*(sigma^2)))*((RobotinoPos(1)-Stationen(1,x))/(sigma^2));
SVY(x)= -K*exp(-((RobotinoPos(1)-Stationen(1,x))^2+(RobotinoPos(2)-Stationen(2,x))^2)/(2*(sigma^2)))*((RobotinoPos(2)-Stationen(2,x))/(sigma^2));
end
K=300;
sigma=100; %% mal schauen ob so gut
for x=5:6 %% Ladestation
SVX(x)= -K*exp(-((RobotinoPos(1)-Stationen(1,x))^2+(RobotinoPos(2)-Stationen(2,x))^2)/(2*(sigma^2)))*((RobotinoPos(1)-Stationen(1,x))/(sigma^2));
SVY(x)= -K*exp(-((RobotinoPos(1)-Stationen(1,x))^2+(RobotinoPos(2)-Stationen(2,x))^2)/(2*(sigma^2)))*((RobotinoPos(2)-Stationen(2,x))/(sigma^2));
end
%Zielvektor
K=0.7;%=0.5;
if (RobotinoPos(1)~=ZielPos(1)) && (RobotinoPos(2)~=ZielPos(2))  %%Ziel
    ZVX = K*(RobotinoPos(1)-ZielPos(1))/sqrt((RobotinoPos(1)-ZielPos(1))^2 +(RobotinoPos(2)-ZielPos(2))^2);
    ZVY = K*(RobotinoPos(2)-ZielPos(2))/sqrt((RobotinoPos(1)-ZielPos(1))^2 +(RobotinoPos(2)-ZielPos(2))^2);
else
    ZVX=0;
    ZVY=0;
end

%Robtino Stoervektoren
%K=25 im Fifo

RVX=zeros([1 4]);
RVY=zeros([1 4]);
for x=1:4
if (RobotinoFaehrt(x) == 1) && (RobotinoPos(2)> 500)
K=1300;%K=1000;
sigma=240;
elseif (RobotinoPos(2)> 2500)
K=700;%500
sigma=200;
elseif (RobotinoPos(2)< 2500)
K=1000;%700
sigma=200;
end
RVX(x)=-K*exp(-((RobotinoPos(1)-StoerPos((x*3)-2))^2+(RobotinoPos(2)-StoerPos((x*3)-1))^2)/(2*(sigma^2)))*((RobotinoPos(1)-StoerPos((x*3)-2))/(sigma^2));
RVY(x)=-K*exp(-((RobotinoPos(1)-StoerPos((x*3)-2))^2+(RobotinoPos(2)-StoerPos((x*3)-1))^2)/(2*(sigma^2)))*((RobotinoPos(2)-StoerPos((x*3)-1))/(sigma^2));
end

%Infrarot Einflussvektor
K=600;%500;
sigma=250;
IRVX=zeros([1 9]);
IRVY=zeros([1 9]);
for x=1:9
    if(isnan(IRWerte(1,x))==0)||(isnan(IRWerte(2,x))==0)
       if (RobotinoPos(2)> 500)
    IRVX(x)=-K*exp(-((RobotinoPos(1)-IRWerte(1,x))^2+(RobotinoPos(2)-IRWerte(2,x))^2)/(2*(sigma^2)))*((RobotinoPos(1)-IRWerte(1,x))/(sigma^2));
    IRVY(x)=-K*exp(-((RobotinoPos(1)-IRWerte(1,x))^2+(RobotinoPos(2)-IRWerte(2,x))^2)/(2*(sigma^2)))*((RobotinoPos(2)-IRWerte(2,x))/(sigma^2));
       else
    IRVX=0;
    IRVY=0;
       end
    else
    IRVX(x)=0;
    IRVY(x)=0;
    end
end


 
K=0.4; %Steigung der schrägen
x=RobotinoPos(1);
y=RobotinoPos(2);
x_test=0;
y_test=0;
VektorX=0;
VektorY=0;
%% Einteilung des Vektorbereichs in verschidene Zonen
%%Einbahnstraßen hinter und neben den Stationen
 if (x >601) && (x<=5301) && (y>2501) && (y<=3201)
    Zone=4;
elseif (x >2751) && (x<=5501) && (y>3201)
    Zone=1;
elseif (x > 601) && (x<=2751) && (y>3201)
    Zone=2;
 elseif (x<=601) && (y>2001)%% y auf 2001 von 2501
     Zone=3;  
 elseif (x >5001) && (y>2501) && (AlteZone==1 || AlteZone==5)
     Zone=5;
 else
     Zone=0;
 end

KE=1000;
sigma=50;
Parabel=1000;
 if Zone == 0 % Fahrbereich
     if (x <= 5500) && (y <= 2500)
         x_test=(1/sigma)*KE*exp(-x/sigma);
         y_test=(-1/sigma)*KE*exp((y-2500)/sigma);
     elseif (x > 5500) && (y <= 2500)
         x_test=(1/sigma)*KE*exp((-(x-5500)+(y-2500))/sigma);
         y_test=(-1/sigma)*KE*exp((-(x-5500)+(y-2500))/sigma);
     elseif (x > 5500) && (y > 2500)
         x_test=(1/sigma)*KE*exp(-(x-5500)/sigma);
         y_test=(-1/sigma)*KE*exp((y-3600)/sigma);
     end
 MVX=x_test+(-1/sigma)*KE*exp((x-7400)/sigma);
 MVY=y_test+(1/sigma)*KE*exp(-y/sigma);
 
 VektorX=sum(SVX(5:6))+sum(RVX)+ZVX+sum(IRVX)-MVX;
 VektorY=sum(SVY(5:6))+sum(RVY)+ZVY+sum(IRVY)-MVY;
 elseif Zone == 1 %Rinne nach rechts weg
     MVX=K; %Konstante Steigung
     MVY=-2*(y-3500)/Parabel; % Parabel abgeleitet
 VektorX=sum(RVX)-MVX;
 VektorY=sum(RVY)-MVY;
 elseif Zone == 2 %Rinne nach links weg
     MVX=-K; %Konstante Steigung
     MVY=-2*(y-3500)/Parabel; % Parabel abgeleitet
      VektorX=sum(RVX)-MVX;
      VektorY=sum(RVY)-MVY;
 elseif Zone == 3 %Rinne nach unten weg
     MVX=-2*(x-300)/Parabel; %Konstante Steigung
     MVY=-K; % Parabel abgeleitet
     VektorX=sum(RVX)+sum(IRVX)-MVX;
     VektorY=sum(RVY)+sum(IRVY)-MVY;
 elseif Zone == 5 %Rinne vorne weg
     MVX=-2*(x-5500)/Parabel; %Konstante Steigung
     MVY=-K; % Parabel abgeleitet
     VektorX=sum(RVX)+sum(IRVX)-MVX;
     VektorY=sum(RVY)+sum(IRVY)-MVY;
 else 
     MVX=0;
     MVY=K;
      VektorX=sum(RVX)+sum(SVX(1:4))-MVX;
      VektorY=sum(RVY)+sum(SVY(1:4))-MVY;
 end  
      Vektor(1)=VektorX;
      Vektor(2)=VektorY;
 end

== matlab function Simulation_Robotinos/Bahnplanung3/Vektorbrbegrenzungberchnen1 ==
  data: Vektor_In input; IRDaten input; Vektor output; Transportbereich_aktiv input; RobPos input; FilterIN input; Filter output
function [Vektor,Filter] = fcn(Vektor_In,IRDaten,Transportbereich_aktiv,RobPos,FilterIN)
Vektor=zeros([1 2]);
Filter=zeros([10 2]);
if (Transportbereich_aktiv==1) && (RobPos(1)>=0) && (RobPos(2)>=0)
    

 Filter(1,1)=Vektor_In(1);
 Filter(1,2)=Vektor_In(2);
 for x=1:9
     Filter(x+1,1)=FilterIN(x,1);
     Filter(x+1,2)=FilterIN(x,2);     
 end
 Vektor(1) =sum(Filter(:,1))/10;
 Vektor(2) =sum(Filter(:,2))/10;
 
 %Vektor(1) = Vektor_In(1);
 %Vektor(2) = Vektor_In(2);
 for x=1:9
if  (isnan(IRDaten(1,x))==0) && (IRDaten(1,x) <= 150)
    for x=1:2
    K=0.1; %Begrenzung langsame Zone
        if  Vektor(x)> K
            Vektor(x) = K;
        elseif Vektor(x) <-K
            Vektor(x)=-K;
        end
    end
end
 end
if (RobPos(2)<500)||(RobPos(2)>2300)
    for x=1:2
    K=0.3; %Begrenzung langsame Zone
        if  Vektor(x)> K
            Vektor(x) = K;
        elseif Vektor(x) <-K
            Vektor(x)=-K;
        end
    end
else
    for x=1:2
    K=0.7; %Begrenzung schnelle Zone
        if  Vektor(x)> K
            Vektor(x) = K;
        elseif Vektor(x) <-K
            Vektor(x)=-K;
        end
    end
end
end

== stateflow chart Simulation_Robotinos/Bahnplanung4/Auftrags_Koordination ==
  settings: updateMethod=DISCRETE  sampleTime=dt
  state Auftragskoordination
    state WerkstueckAufgenommen
      entry:Werkstueck=1,
      AktuellesZiel=ZielPos,
      Bearbeitet=1;
    state WerkstueckAbgelegt
      entry:Werkstueck=0,
      AktuellesZiel=ZielPos,
      Bearbeitet=1;
    state KeinWerkstueckAufgenommen
      entry:Werkstueck=0,
      AktuellesZiel=WerkstueckPos,
      Bearbeitet=1;
    state AufAuftragWarten
      entry:Werkstueck=0,
      AktuellesZiel=100
      Bearbeitet=0;
    state Laden
      entry:Werkstueck=0,
      AktuellesZiel=90,
      Bearbeitet=1;
    state Ladenabgeschlossen
      entry:Werkstueck=0,
      AktuellesZiel=90,
      Bearbeitet=1;
    WerkstueckAufgenommen -> WerkstueckAufgenommen [order 1] : [Fehler==3]
    WerkstueckAufgenommen -> WerkstueckAbgelegt [order 3] : [Werkstueckerkannt==0 && Transportbereich==0]
    KeinWerkstueckAufgenommen -> WerkstueckAufgenommen [order 1] : [Werkstueckerkannt==1 && Transportbereich==1]
    WerkstueckAufgenommen -> AufAuftragWarten [order 2] : [Fehler==2  && Transportbereich==1]
    (default) -> AufAuftragWarten
    WerkstueckAbgelegt -> AufAuftragWarten : [Werkstueckerkannt==0 && Transportbereich==1]
    KeinWerkstueckAufgenommen -> AufAuftragWarten [order 2] : [Fehler==1&& Transportbereich==1]
    AufAuftragWarten -> KeinWerkstueckAufgenommen [order 1] : [NeuerAuftrag ==1 && WerkstueckPos< 80 && Fehler==0]
    AufAuftragWarten -> Laden [order 2] : [NeuerAuftrag ==1 && WerkstueckPos>= 80]
    Ladenabgeschlossen -> AufAuftragWarten : [Transportbereich==1]
    Laden -> Ladenabgeschlossen : [Status==4]
  data: NeuerAuftrag input; WerkstueckPos input; ZielPos input; AktuellesZiel output; Werkstueck output; Werkstueckerkannt input; Transportbereich input; Bearbeitet output; Status input; Fehler input

== matlab function Simulation_Robotinos/Bahnplanung4/Fehler_Merker ==
  data: Fehler_IN input; Reset input; Transportbereich input; Werkstueckerkannt input; Werkstueck input; Fehler_OUT output; Fehler_alt input
function Fehler_OUT       = fcn(Fehler_IN ,Reset, Transportbereich, Werkstueckerkannt,Werkstueck, Fehler_alt)
if Reset == 1 || Fehler_IN ~= 0
    Fehler_OUT=Fehler_IN;
else
    if Transportbereich == 1 && Werkstueckerkannt~=1 && Werkstueck == 1
        Fehler_OUT = 2;
    else
       Fehler_OUT=Fehler_alt; 
    end 
end
end

== stateflow chart Simulation_Robotinos/Bahnplanung4/Fifo Steuerung/Fifo ==
  settings: updateMethod=DISCRETE  sampleTime=dt
  state FIFOStationen
    state Auftrag_Roboter_1
    state Zielbereich_untersuchen
      entry:
      ersterFifo=floor(Zielstation/2)*3+2*mod(Zielstation,2)+1;
    state Fifo_doppelt_besetzt
      entry:
      dritterFifo=floor(Zielstation/2)*3+2-2*mod(Zielstation,2)+1,
      Fifo=3;
    state Fifo_einfachbesetzt1
      entry:
      zweiterFifo=floor(Zielstation/2)*3+1+1,
      Fifo=2;
    state Fifo_voll
      entry:
      Fifo=4;
    state Fifo_frei
      entry:
      Fifo=1;
    state Uebergabepunkt_gleich_Zielpunkt
      entry:
      Fifo=0;
    (default) -> Auftrag_Roboter_1
    Auftrag_Roboter_1 -> Zielbereich_untersuchen : [Zielposition>-1]
    Zielbereich_untersuchen -> Fifo_einfachbesetzt1 [order 1] : [(FifoArray(ersterFifo)~=0)| (FifoArray(ersterFifo)==0 & StationArray(Zielstation+1)~=0) ]
    Uebergabepunkt_gleich_Zielpunkt -> Zielbereich_untersuchen
    Zielbereich_untersuchen -> Uebergabepunkt_gleich_Zielpunkt [order 2]
    Fifo_einfachbesetzt1 -> Fifo_doppelt_besetzt [order 1] : [(FifoArray(zweiterFifo)~=0)]
    Fifo_doppelt_besetzt -> Fifo_voll [order 2] : [(FifoArray(dritterFifo)~=0)]
    Fifo_einfachbesetzt1 -> Fifo_frei [order 2] : [FifoArray(ersterFifo)==0]
    Fifo_doppelt_besetzt -> Fifo_einfachbesetzt1 [order 1] : [FifoArray(zweiterFifo)==0]
    Fifo_frei -> Uebergabepunkt_gleich_Zielpunkt : [ StationArray(Zielstation+1)==0]
    Fifo_voll -> Fifo_doppelt_besetzt : [FifoArray(dritterFifo)==0]
  state Wartebereich
    entry: Fifo=4;
  state Ladestation
    entry: Fifo=0;
  state Ladestation1
    entry: Fifo=4;
  FIFOStationen -> FIFOStationen [order 1] : [after(10000, tick)]
  (default) -> Wartebereich
  Wartebereich -> FIFOStationen [order 1] : [Zielstation<8]
  FIFOStationen -> Wartebereich [order 2] : [Zielstation==10]
  Ladestation -> Wartebereich [order 1] : [Zielstation==10]
  Wartebereich -> Ladestation [order 2] : [Zielstation>=8 & Zielstation<10]
  Ladestation -> FIFOStationen [order 2] : [Zielstation<8]
  FIFOStationen -> Ladestation [order 3] : [Zielstation>=8 & Zielstation<10]
  Ladestation -> Ladestation1 [order 3] : [Ladenarray(1)~=0]
  Ladestation1 -> Ladestation : [Ladenarray(1)==0]
  data: FifoArray input; Zielposition input; Zielstation input; Fifo output; StationArray input; dritterFifo local; zweiterFifo local; ersterFifo local; Ladenarray input

== matlab function Simulation_Robotinos/Bahnplanung4/Fifo Steuerung/Globale Markierung1 ==
  data: StationArray1 output; Robbi input; FifoArray input; FifoArray1 output; LadeArray1 output; LadeArray input
function [StationArray1,FifoArray1,LadeArray1]= fcn(Robbi,FifoArray,LadeArray)
X=zeros([1 4]);
Y=zeros([1 4]);
X=[Robbi(1) Robbi(4) Robbi(7) Robbi(10)];
Y=[Robbi(2) Robbi(5) Robbi(8) Robbi(11)];
FifoArray1=zeros([1 12]);
FifoArray1=FifoArray(1:12);
StationArray1=zeros([1 8]);
LadeArray1=zeros([1 2]);
LadeArray1=LadeArray(1:2);
N=zeros([1 4]);
S=zeros([1 4]);
L=zeros([1 4]);
  for n= 1 : 1 : 4
    L(n)=round((Y(n)-2592)/500)+1;
    N(n)=round((X(n)-703)/425)+1;   % Berechnung in welchem Fifo der Roboter sich befindet
    S(n)=round((X(n)-900)/560)+1;   %Berechnung in welcher Station der Roboter sich befindet
     if (X(n)<=6000 || X(n)>6500)
        for i=1:2
            if LadeArray1(i)==n
                LadeArray1(i)=0;
            end
        end
     end
    if (X(n)>6000 && X(n)<=6500 && Y(n)>2300 && Y(n)<=3300 && L(n)<=2 && L(n)>0)
        LadeArray1(1)=n;
        LadeArray1(2)=n;
    end  
   
    for i=1:8
          if StationArray1(i)==n
                StationArray1(i)=0;
          end
    end
    if (Y(n)>2000 && Y(n)<3300 && X(n)<5100 && S(n)<=8 && S(n)>0) %% Setzen der Stationspos.
         for i=1:12
            if FifoArray1(i)==n
                FifoArray1(i)=0;
            end
         end
       
        StationArray1(S(n))=n;
    end
    if (Y(n)<450 && X(n)>100 && X(n)<6000 && N(n)<=12 && N(n)>0) %% Setzten der aktuellen Fifo Pos
        for i=1:12
            if FifoArray1(i)==n
                FifoArray1(i)=0;
            end
        end
            FifoArray1(N(n))=n;
    end  
    if (X(n)>6000 && Y(n)<2000)%%Rücksetzen de4r FIFOs auf Warteposition
        for i=1:12
            if FifoArray1(i)==n
                FifoArray1(i)=0;
            end
        end
    end
  end
end

== matlab function Simulation_Robotinos/Bahnplanung4/Fifo Steuerung/Positionszuweisung ==
  data: Fifo input; Zielstation input; Endposition output; RoboterID input
function Endposition = fcn(Fifo,Zielstation,RoboterID)
Endposition=zeros([1 2]);

WartepositionX= [6200 6800 7200 7200 7200]; %[7200 6800 7200 6200 7200];
WartepositionY= [250 250 550 1150 1750];    %[550 250 1150 250 1750];

StationvorneX=[853 1361 2058 2559 3256 3762 4448 4953 5965 5965];
StationvorneY=[2300 2300 2300 2300 2300 2300 2300 2300 3080 2593];
%Stationhinten=[856 1364 2059 2560 3259 3763 4451 4958];

ersterFifo=floor(Zielstation/2)*3+2*mod(Zielstation,2);
zweiterFifo=floor(Zielstation/2)*3+1;
dritterFifo=floor(Zielstation/2)*3+2-2*mod(Zielstation,2);

if Fifo==0
    Endposition(1)=StationvorneX(Zielstation+1);
    Endposition(2)=StationvorneY(Zielstation+1);
    else if Fifo==1
        Endposition(1)= ersterFifo*425+703;
        Endposition(2)= 250;
       
    else if Fifo==2
            Endposition(1)= zweiterFifo*425+703;
            Endposition(2)= 250;
        
    else if Fifo==3
            Endposition(1)= dritterFifo*425+703;
            Endposition(2)= 250;
            else
            Endposition(2)= WartepositionY(RoboterID);
            Endposition(1)= WartepositionX(RoboterID);
        end
        end
        end
end
end

== matlab function Simulation_Robotinos/Bahnplanung4/Fifo Steuerung/ZielPosSplitten ==
  data: AktuellesZiel input; ZielPos output; Zielstation output
function [ZielPos,Zielstation]= fcn(AktuellesZiel)
ZielPos=mod(AktuellesZiel,10);
Zielstation=round(AktuellesZiel/10);

== matlab function Simulation_Robotinos/Bahnplanung4/Fifo Steuerung/ZielStation_Erreicht ==
  data: Erreicht output; AktuellePos input; Zielpos input
function Erreicht = fcn(AktuellePos,Zielpos)
Abstand=sqrt((AktuellePos(1)-Zielpos(1))^2+(AktuellePos(2)-Zielpos(2))^2);
%S=round((X-900)/560);
if AktuellePos(2) >2000 && Abstand < 150
    Erreicht=1;
else
    Erreicht=0;
end
end
